simulink model "model_trapezoidal_gust"  (R2020b)
settings: Solver=VariableStepAuto  StartTime=0.0  StopTime=10.0  RelTol=1e-3
undefined symbols (not defined in the file or in its folder): trapezoidal_gust
settings Model: Creator=C:\Users\Dogukan  LastModifiedBy=C:\Users\Dogukan

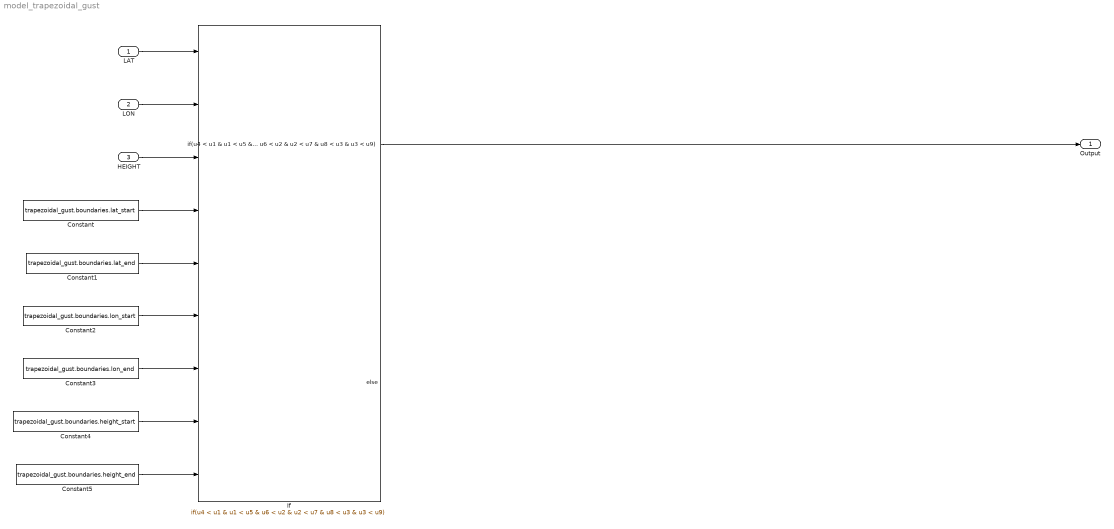
== system model_trapezoidal_gust ==
  LAT : Inport
  LON : Inport  Port=2
  HEIGHT : Inport  Port=3
  Constant : Constant  Value=trapezoidal_gust.boundaries.lat_start
  Constant1 : Constant  Value=trapezoidal_gust.boundaries.lat_end
  Constant2 : Constant  Value=trapezoidal_gust.boundaries.lon_start
  Constant3 : Constant  Value=trapezoidal_gust.boundaries.lon_end
  Constant4 : Constant  Value=trapezoidal_gust.boundaries.height_start
  Constant5 : Constant  Value=trapezoidal_gust.boundaries.height_end
  If : If  NumInputs=9  IfExpression=u4 < u1 & u1 < u5 & u6 < u2 & u2 < u7 & u8 < u3 & u3 < u9
  Output : Outport
  wires:
  Constant5/1 -> If/9
  Constant/1 -> If/4
  Constant3/1 -> If/7
  HEIGHT/1 -> If/3
  LAT/1 -> If/1
  Constant2/1 -> If/6
  Constant4/1 -> If/8
  LON/1 -> If/2
  Constant1/1 -> If/5
  If/1 -> Output/1
